simulink model "Thermal_Tension_Transfer_Register"  (R2021b)
settings: Solver=ode4  StartTime=0.0  StopTime=1000  FixedStep=0.1  RelTol=1e-3
undefined symbols (not defined in the file): A, E1eq, E1t, ep1eq, L1, tau1, v00, v10
settings Model: Creator=ZeroHertz  LastModifiedBy=Zerohertz
settings GRTTargetCC: DynamicStringBufferSize=25600

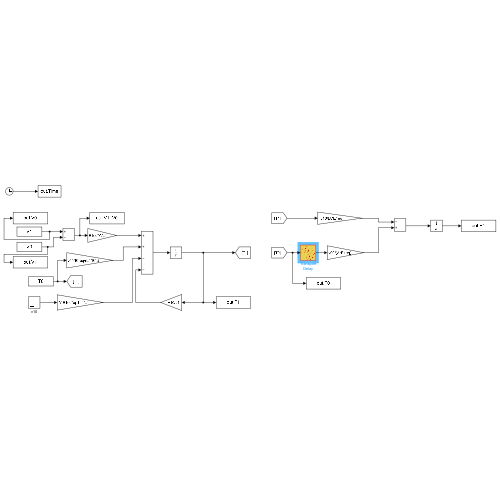
[thumbnail: Simulink's stored preview of the top-level diagram]
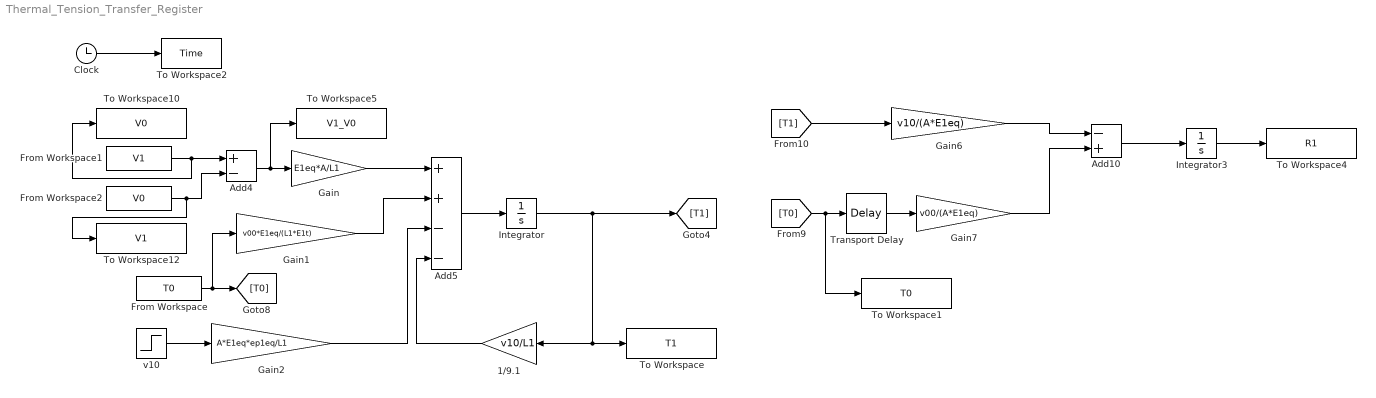
== system Thermal_Tension_Transfer_Register ==
  1/9.1 : Gain  Gain=v10/L1
  Add10 : Sum  Inputs=-+
  Add4 : Sum  Inputs=+-
  Add5 : Sum  Inputs=++--
  Clock : Clock
  From Workspace : FromWorkspace  VariableName=T0
  From Workspace1 : FromWorkspace  VariableName=V1
  From Workspace2 : FromWorkspace  VariableName=V0
  Gain : Gain  Gain=E1eq*A/L1
  Gain1 : Gain  Gain=v00*E1eq/(L1*E1t)
  Gain2 : Gain  Gain=A*E1eq*ep1eq/L1
  Gain6 : Gain  Gain=v10/(A*E1eq)
  Gain7 : Gain  Gain=v00/(A*E1eq)
  Integrator : Integrator
  Integrator3 : Integrator
  To Workspace : ToWorkspace  VariableName=T1  SampleTime=-1
  To Workspace1 : ToWorkspace  VariableName=T0  SampleTime=-1
  To Workspace10 : ToWorkspace  VariableName=V0  SampleTime=-1
  To Workspace12 : ToWorkspace  VariableName=V1  SampleTime=-1
  To Workspace2 : ToWorkspace  VariableName=Time  SampleTime=-1
  To Workspace4 : ToWorkspace  VariableName=R1  SampleTime=-1
  To Workspace5 : ToWorkspace  VariableName=V1_V0  SampleTime=-1
  Transport Delay : TransportDelay  DelayTime=tau1  BufferSize=25600
  v10 : Step  Time=0  Before=v10  After=v10  SampleTime=0
  wires:
  Gain/1 -> Add5/1
  Gain1/1 -> Add5/2
  1/9.1/1 -> Add5/4
  Clock/1 -> To Workspace2/1
  From Workspace1/1 -> To Workspace10/1, Add4/1
  Add4/1 -> To Workspace5/1, Gain/1
  From Workspace/1 -> Gain1/1, [T0]
  Integrator/1 -> 1/9.1/1, To Workspace/1, [T1]
  From Workspace2/1 -> To Workspace12/1, Add4/2
  Add5/1 -> Integrator/1
  Integrator3/1 -> To Workspace4/1
  [T1] -> Gain6/1
  Gain6/1 -> Add10/1
  Gain7/1 -> Add10/2
  Transport Delay/1 -> Gain7/1
  [T0] -> To Workspace1/1, Transport Delay/1
  Add10/1 -> Integrator3/1
  v10/1 -> Gain2/1
  Gain2/1 -> Add5/3
